simulink model "Copter_Plane_h2g_V10g"  (R2020b)
(part 3 of 5)

  Delay5/1 -> Scope100/2, Location_offset1/3(ofs_east)
  Gain26/1 -> Scope170/2
  Data Store Read116/1 -> MATLAB Function1/4(k_elevator), Scope66/1
  [DCM_be] -> Inertial to Body4/1
  Gain49/1 -> Scope67/1
  Demux20/3 -> MATLAB Function1/7(wz)
  Constant33/1 -> Data Store Write48/1
  Data Store Read45/1 -> Scope176/2
  Demux47/1 -> Atan3/2
  Data Store Read54/1 -> Gain47/1
  Gain40/1 -> Scope72/1
  Demux10/2 -> Data Store Write57/1
  Gain37/1 -> Scope68/1
  Demux15/2 -> Scope155/2
  Data Store Read/1 -> Scope2/1
  Gain33/1 -> Scope178/1
  Data Store Read34/1 -> Scope170/1
  Demux47/2 -> Atan3/1
  Gain42/1 -> Scope28/1, Scope87/1
  Demux41/2 -> Delay5/1
  Atan4/1 -> [yaw_w]
  Demux42/1 -> Scope58/1
  Gain46/1 -> Scope114/2
  Constant14/1 -> Data Store Write55/1
  Demux10/3 -> Data Store Write58/1
  Data Store Read44/1 -> Scope176/1
  Delay4/1 -> Location_offset1/2(ofs_north), Scope99/2
  6DOF (Euler Angles)2/3(Euler) -> [euler]
  Mux4/1 -> Sum1/2
  Constant26/1 -> Data Store Write34/1
  Data Store Read58/1 -> Scope126/1
  Data Store Read150/1 -> Scope83/3  "I"
  Data Store Read79/1 -> Scope83/2, Scope3/1  "D"
  Data Store Read1/1 -> Scope83/1, Scope54/1  "P"
  Data Store Read151/1 -> Scope83/4
  Gain3/1 -> Scope81/1
  Data Store Read83/1 -> Gain3/1
  Add4/1 -> Gain85/1
  Data Store Read149/1 -> Gain79/1
  Gain84/1 -> Add3/1
  Data Store Read5/1 -> Scope6/1
  Data Store Read8/1 -> Scope7/1
  Gain76/1 -> Scope9/1
  Data Store Read144/1 -> Gain76/1
  Data Store Read11/1 -> Gain83/1
  Data Store Read147/1 -> Gain78/1
  Gain77/1 -> Scope9/3
  Add/1 -> Gain84/1
  Gain83/1 -> Scope8/1, Add/1  "P"
  Gain79/1 -> Scope10/3
  Data Store Read166/1 -> Add4/1, Add3/2
  Gain85/1 -> Scope8/4
  Data Store Read148/1 -> Scope10/2
  Gain72/1 -> Scope8/2, Add/2  "D"
  Data Store Read10/1 -> Scope8/3, Add/3  "I"
  Data Store Read145/1 -> Scope9/2
  Data Store Read146/1 -> Gain77/1
  Data Store Read167/1 -> Add4/2, Scope78/2
  Gain78/1 -> Scope10/1
  Data Store Read9/1 -> Gain72/1
  Data Store Read4/1 -> Scope5/1
  Add3/1 -> Scope78/1
  Demux2/2 -> Scope12/2
  Data Store Read13/1 -> Demux2/1
  Demux1/3 -> Scope13/1
  Demux1/2 -> Scope12/1
  Demux1/1 -> Scope11/1
  Demux2/1 -> Scope11/2
  Demux1/4 -> Scope14/1
  Demux2/4 -> Scope14/2
  Demux2/3 -> Scope13/2
  MATLAB Function/1(PWM_n) -> Demux1/1
  Data Store Read12/1 -> MATLAB Function/1(PWM)
  Data Store Read14/1 -> Scope16/2
  Demux/2 -> Scope16/1
  Data Store Read2/1 -> Scope4/1
  Data Store Read3/1 -> Scope20/1
  Data Store Read15/1 -> Scope21/1
  Data Store Read16/1 -> MATLAB Function1/10(V)
  Add8/1 -> Gain/1
  MATLAB Function1/1(F) -> Add5/1, Scope26/1
  Subsystem1/1(Motor Forces) -> Scope23/1, Add5/2
  MATLAB Function1/2(M) -> Add7/1, Scope27/1
  Subsystem1/2(Motor Torques) -> Add7/2, Demux3/1, Scope19/1
  Divide/1 -> Scope41/1
  Constant2/1 -> Add8/2
  Gain/1 -> Sqrt/1
  Sqrt/1 -> Subsystem1/4(Motor Commands)
  ? -> Subsystem1/1(Vb), Scope42/1
  ? -> Subsystem1/3(pqr), Scope43/1
  Transpose/1 -> Add8/1
  Data Store Read18/1 -> Scope22/1
  Data Store Read19/1 -> Scope24/2
  Demux3/2 -> Scope24/1
  Atan1/1 -> [theta]
  [theta] -> Gain5/1
  Data Store Read20/1 -> Gain4/1
  Gain5/1 -> Scope28/3
  Gain4/1 -> Scope28/2
  Hypot2/1 -> Atan1/2, Data Store Write32/1
  Gain6/1 -> Atan1/1
  Repeating Sequence/1 -> Divide/1, Scope29/1
  Constant3/1 -> Divide/2
  Data Type Conversion9/1 -> ?  "accel_y"
  Bus Selector2/3 -> Data Type Conversion7/1  "<gyro_z>"
  input_euler_angle_roll_pitch_euler_rate_yaw4/4(k_aileronL_o) -> Bus Assignment/5  "k_rudderL"
  input_euler_angle_roll_pitch_euler_rate_yaw4/3(k_rudder_o) -> Bus Assignment/4  "k_rudder"
  Bus Selector/2 -> Data Store Write2/4  "<curLLA>"
  Bus Selector2/2 -> Data Type Conversion6/1  "<gyro_y>"
  Bus Selector2/6 -> Data Type Conversion10/1  "<accel_z>"
  Bus Selector1/2 -> Data Type Conversion1/1  "<rolld>"
  input_euler_angle_roll_pitch_euler_rate_yaw4/7(pwm_out_o) -> Bus Assignment/8  "pwm_out"
  Bus Selector1/4 -> Data Type Conversion11/1  "<alt>"
  input_euler_angle_roll_pitch_euler_rate_yaw4/8(pwm_tail_o) -> Bus Assignment/9  "pwm_tail"
  Bus Selector2/4 -> Data Type Conversion8/1  "<accel_x>"
  PathModeOut/1 -> Data Store Write2/9  "PathModeOut"
  IMU/1 -> Bus Selector2/1
  plane_mode_in/1 -> plane_mode1/1
  Bus Selector1/1 -> Data Type Conversion/1  "<pitchd>"
  NAVI2CONTROL/1 -> Bus Selector1/1
  input_euler_angle_roll_pitch_euler_rate_yaw4/9(k_flap_o) -> Bus Assignment/10  "k_flap"
  CTRL_remote_ct_st/1 -> algo_remote_ct_st1/1
  input_euler_angle_roll_pitch_euler_rate_yaw4/2(k_elevator_o) -> Bus Assignment/3  "k_elevator"
  TASK_COMMON_OutParam/1 -> Bus Selector/1
  Bus Assignment/1 -> Out1/1
  Constant/1 -> Bus Assignment/1
  Data Type Conversion10/1 -> ?  "accel_z"
  input_euler_angle_roll_pitch_euler_rate_yaw4/6(tail_tilt_o) -> Bus Assignment/7  "tail_tilt"
  Bus Selector3/2 -> Data Type Conversion4/1  "<EAS2TAS_Algo>"
  Bus Selector2/5 -> Data Type Conversion9/1  "<accel_y>"
  Data Type Conversion/1 -> Data Store Write2/5  "pitchd"
  Data Type Conversion5/1 -> ?  "gyro_x"
  input_euler_angle_roll_pitch_euler_rate_yaw4/5(k_aileronR_o) -> Bus Assignment/6  "k_rudderR"
  EAS_Algo/1 -> Bus Selector3/1  "EAS_Algo"
  Data Type Conversion3/1 -> Data Store Write2/1  "EAS_Algo"
  CTRL_wp/1 -> Data Store Write2/10  "wp_in"
  Bus Selector1/3 -> Data Type Conversion2/1  "<yawd>"
  Data Type Conversion8/1 -> ?  "accel_x"
  Bus Selector/1 -> Data Store Write2/3  "<curVelNED>"
  CTRL_dbg_param/1 -> algo_dbg_param1/1
  input_euler_angle_roll_pitch_euler_rate_yaw4/1(k_alieron_o) -> Bus Assignment/2  "k_aileron"
  Data Type Conversion7/1 -> ?  "gyro_z"
  Data Type Conversion2/1 -> Data Store Write2/7  "yawd"
  Bus Selector2/1 -> Data Type Conversion5/1  "<gyro_x>"
  Data Type Conversion11/1 -> Data Store Write2/8  "NAV_alt"
  Data Type Conversion1/1 -> Data Store Write2/6  "rolld"
  Data Type Conversion6/1 -> ?  "gyro_y"
  Data Type Conversion4/1 -> Data Store Write2/2  "EAS2TAS_Algo"
  Bus Selector3/1 -> Data Type Conversion3/1  "<airspeed_indicate>"
  Data Store Read21/1 -> Scope30/1
  Data Store Read21/8 -> Scope37/1
  Data Store Read21/6 -> Scope35/1
  Data Store Read21/2 -> Scope31/1
  Data Store Read21/7 -> Scope36/1
  Data Store Read21/5 -> Scope34/1
  Data Store Read21/4 -> Scope33/1
  Data Store Read21/3 -> Scope32/1
  Data Store Read21/9 -> Scope38/1
  Data Store Read21/10 -> Scope39/1
  Clock/1 -> Data Store Write5/1
  Data Store Read17/1 -> Mux/1
  Data Store Read32/1 -> Transpose/1
  Constant4/1 -> Mux/2
  Data Store Read22/1 -> Gain7/1
  Data Store Read23/1 -> Gain8/1
  Data Store Read26/1 -> Gain9/1
  Data Store Read24/1 -> Gain10/1
  Gain7/1 -> Scope44/1
  Gain8/1 -> Scope44/2
  Gain9/1 -> Scope45/1
  Gain10/1 -> Scope45/2
  Data Store Read27/1 -> Gain11/1
  Data Store Read25/1 -> Gain12/1
  Gain11/1 -> Scope46/1
  Gain12/1 -> Scope46/2
  Data Store Read29/1 -> Gain15/1
  Data Store Read31/1 -> Gain17/1
  Gain17/1 -> Scope47/1
  Data Store Read28/1 -> Gain13/1
  Gain16/1 -> Scope47/2
  Data Store Read30/1 -> Gain16/1
  Gain13/1 -> Scope48/2
  Gain15/1 -> Scope48/1
  Data Store Read33/1 -> Demux5/1
  Data Store Read35/1 -> Demux6/1
  Demux6/1 -> Scope50/1
  Demux5/1 -> Scope50/2
  Demux6/2 -> Scope51/1
  Demux5/2 -> Scope51/2
  Data Store Read47/1 -> Demux7/1
  Data Store Read49/1 -> Demux8/1
  Demux7/1 -> Scope52/2
  Demux8/1 -> Scope52/1
  Demux8/2 -> Scope53/1
  Demux7/2 -> Scope53/2
  Data Store Read80/1 -> MATLAB Function4/1(x_cmss)
  Data Store Read61/1 -> MATLAB Function3/2(y_cmss)
  Data Store Read51/1 -> MATLAB Function2/2(y_cmss)
  Data Store Read52/1 -> MATLAB Function3/1(x_cmss)
  Data Store Read73/1 -> MATLAB Function6/2(y_cmss)
  Data Store Read78/1 -> MATLAB Function5/2(y_cmss)
  Data Store Read77/1 -> MATLAB Function5/1(x_cmss)
  MATLAB Function4/1(forward) -> Scope55/2, Scope62/1
  Data Store Read72/1 -> MATLAB Function6/1(x_cmss)
  Data Store Read76/1 -> Gain18/1
  Data Store Read102/1 -> MATLAB Function2/1(x_cmss)
  Gain18/1 -> Tan/1
  MATLAB Function2/1(forward) -> Scope61/1
  MATLAB Function3/1(forward) -> Scope84/1, Scope57/1, Scope55/1
  MATLAB Function6/1(forward) -> Scope57/2, Scope56/1, Scope91/1, Scope89/1, Scope62/2
  Data Store Read81/1 -> MATLAB Function4/2(y_cmss)
  MATLAB Function5/1(forward) -> Scope61/2
  Tan/1 -> Gain23/1
  Gain23/1 -> Gain24/1
  Gain24/1 -> Scope56/2
  Gain27/1 -> Gain50/1
  Gain25/1 -> Tan1/1
  Data Store Read90/1 -> Gain25/1
  Tan1/1 -> Gain27/1
  Data Store Read91/1 -> Gain20/1
  Gain20/1 -> Tan2/1
  Gain50/1 -> Divide1/2
  Tan2/1 -> Divide1/1
  Divide1/1 -> Scope64/2
  Data Store Read75/1 -> Gain19/1
  Gain21/1 -> Scope90/2, Scope79/1
  Gain19/1 -> Scope77/2, Scope70/1
  Data Store Read98/1 -> Scope77/1
  Data Store Read99/1 -> Gain21/1
  Data Store Read101/1 -> Scope82/1
  Data Store Read100/1 -> Scope82/2
  Data Store Read103/1 -> MATLAB Function12/1(x_cmss)
  Data Store Read104/1 -> MATLAB Function12/2(y_cmss)
  MATLAB Function12/1(forward) -> Scope84/2
  Demux11/1 -> Gain51/1
  [accelg] -> Inertial to Body1/2
  Inertial to Body1/1 -> Demux11/1
  Data Store Read87/1 -> MATLAB Function8/2(y_cmss)
  Data Store Read93/1 -> MATLAB Function13/2(y_cmss)
  Data Store Read89/1 -> MATLAB Function9/2(y_cmss)
  Data Store Read115/1 -> MATLAB Function10/1(x_cmss)
  MATLAB Function10/2(right) -> Scope40/2, Scope74/1
  Data Store Read153/1 -> MATLAB Function10/2(y_cmss)
  MATLAB Function13/2(right) -> Scope74/2, Scope59/1, Scope64/1, Scope63/2
  Data Store Read84/1 -> MATLAB Function8/1(x_cmss)
  MATLAB Function8/2(right) -> Scope69/2
  Data Store Read92/1 -> MATLAB Function13/1(x_cmss)
  Data Store Read94/1 -> MATLAB Function11/1(x_cmss)
  MATLAB Function7/2(right) -> Scope75/2
  Data Store Read95/1 -> MATLAB Function11/2(y_cmss)
  MATLAB Function9/2(right) -> Scope75/1, Scope63/1, Scope40/1
  Data Store Read86/1 -> MATLAB Function7/2(y_cmss)
  Data Store Read85/1 -> MATLAB Function7/1(x_cmss)
  MATLAB Function11/2(right) -> Scope69/1
  Data Store Read88/1 -> MATLAB Function9/1(x_cmss)
  Data Store Read96/1 -> Gain22/1
  Gain22/1 -> Scope70/2
  Data Store Read155/1 -> Gain55/1
  Gain55/1 -> Scope79/2
  Data Store Read97/1 -> Scope90/1
  Data Store Read82/1 -> Mux6/1
  Data Store Read157/1 -> Mux6/3
  Data Store Read156/1 -> Mux6/2
  Mux6/1 -> Inertial to Body3/2
  Inertial to Body3/1 -> Add6/1, Scope94/1
  Gain53/1 -> Scope59/2
  Gain54/1 -> Scope91/2, Scope104/2
  Data Store Read162/1 -> Mux8/1
  Data Store Read161/1 -> Mux8/2
  Constant8/1 -> Mux8/3
  Mux8/1 -> Selector/1
  Rotation Angles to Direction Cosine Matrix2/1 -> Transpose1/1
  gn1/1 -> Add6/2
  Demux18/1 -> MATLAB Function14/1(x_cmss)
  Demux18/2 -> MATLAB Function14/2(y_cmss)
  MATLAB Function14/2(right) -> Gain53/1
  MATLAB Function14/1(forward) -> Gain54/1
  Gravity in Earth Axes1/1 -> [accel]
  Add6/1 -> Scope101/1, Demux18/1
  Selector/1 -> Rotation Angles to Direction Cosine Matrix2/1
  Transpose1/1 -> Inertial to Body3/1
  Gravity in Earth Axes3/1 -> [accelg]
  Gain51/1 -> Scope104/1, Scope89/2
  Selector1/1 -> Rotation Angles to Direction Cosine Matrix3/1
  Data Store Read154/1 -> Mux2/1
  Constant6/1 -> Mux2/3
  Rotation Angles to Direction Cosine Matrix3/1 -> Transpose2/1
  Data Store Read152/1 -> Mux2/2
  Mux2/1 -> Selector1/1
  Transpose2/1 -> Inertial to Body1/1
  Data Store Read105/1 -> Scope76/1
  Data Store Read158/1 -> MATLAB Function15/1(u)
  MATLAB Function15/1(y) -> Gain56/1
  attitude_error_vector/1 -> Gain29/1
  Gain29/1 -> Display/1
  Data Store Read106/1 -> Gain52/1
  Gain52/1 -> Display2/1
  Gain56/1 -> Display3/1
  rot_body_to_ned/1 -> MATLAB Function16/1(u)
  MATLAB Function16/1(y) -> Gain57/1
  Gain57/1 -> Display4/1
